simulink model "obstacle_detection"  (R2022b)
settings: Solver=VariableStepAuto  StartTime=0.0  StopTime=10.0  RelTol=1e-3
values from neighbouring files (symbols this model uses):
  m = 12    [mpc.m]    (also in mpc_soln.m; qp_soln.m)
  N = 50    [mpc.m]    (also in mpc_caller.m = 20; qp_caller.m = params.N)
  X = [p; reshape(R, [9 1]); v; R'*w]    [mpc_caller.m]    (also in qp_caller.m)
undefined symbols (not defined in the file or in its folder): Y, Z
libraries: sm_lib x269, nesl_utility x117, simulink x2
(part 4 of 5)

== system obstacle_detection/Subsystem11 ==
  PS-Simulink Converter : nesl_utility/PS-Simulink Converter  PhysicalDomain=network_engine_domain  SubClassName=ps_output  LeftPortType=input  RightPortType=output  PseudoPeriodic=off  Frequencies=[]  VectorFormat=inherit  Unit=inherit  AffineConversion=off
  PS-Simulink Converter1 : nesl_utility/PS-Simulink Converter  PhysicalDomain=network_engine_domain  SubClassName=ps_output  LeftPortType=input  RightPortType=output  PseudoPeriodic=off  Frequencies=[]  VectorFormat=inherit  Unit=inherit  AffineConversion=off
  PS-Simulink Converter2 : nesl_utility/PS-Simulink Converter  PhysicalDomain=network_engine_domain  SubClassName=ps_output  LeftPortType=input  RightPortType=output  PseudoPeriodic=off  Frequencies=[]  VectorFormat=inherit  Unit=inherit  AffineConversion=off
  1 : PMIOPort  Side=Left
  2 : PMIOPort  Port=2  Side=Left
  3 : PMIOPort  Port=3  Side=Left
  q : Outport
  w : Outport  Port=2
  t : Outport  Port=3
  wires:
  PS-Simulink Converter2/1 -> t/1
  PS-Simulink Converter1/1 -> w/1
  PS-Simulink Converter/1 -> q/1
  connections:
  3/RConn1 -- PS-Simulink Converter2/LConn1
  2/RConn1 -- PS-Simulink Converter1/LConn1
  1/RConn1 -- PS-Simulink Converter/LConn1

== system obstacle_detection/Subsystem12 ==
  PS-Simulink Converter : nesl_utility/PS-Simulink Converter  PhysicalDomain=network_engine_domain  SubClassName=ps_output  LeftPortType=input  RightPortType=output  PseudoPeriodic=off  Frequencies=[]  VectorFormat=inherit  Unit=inherit  AffineConversion=off
  PS-Simulink Converter1 : nesl_utility/PS-Simulink Converter  PhysicalDomain=network_engine_domain  SubClassName=ps_output  LeftPortType=input  RightPortType=output  PseudoPeriodic=off  Frequencies=[]  VectorFormat=inherit  Unit=inherit  AffineConversion=off
  PS-Simulink Converter2 : nesl_utility/PS-Simulink Converter  PhysicalDomain=network_engine_domain  SubClassName=ps_output  LeftPortType=input  RightPortType=output  PseudoPeriodic=off  Frequencies=[]  VectorFormat=inherit  Unit=inherit  AffineConversion=off
  1 : PMIOPort  Side=Left
  2 : PMIOPort  Port=2  Side=Left
  3 : PMIOPort  Port=3  Side=Left
  q : Outport
  w : Outport  Port=2
  t : Outport  Port=3
  wires:
  PS-Simulink Converter2/1 -> t/1
  PS-Simulink Converter1/1 -> w/1
  PS-Simulink Converter/1 -> q/1
  connections:
  3/RConn1 -- PS-Simulink Converter2/LConn1
  2/RConn1 -- PS-Simulink Converter1/LConn1
  1/RConn1 -- PS-Simulink Converter/LConn1

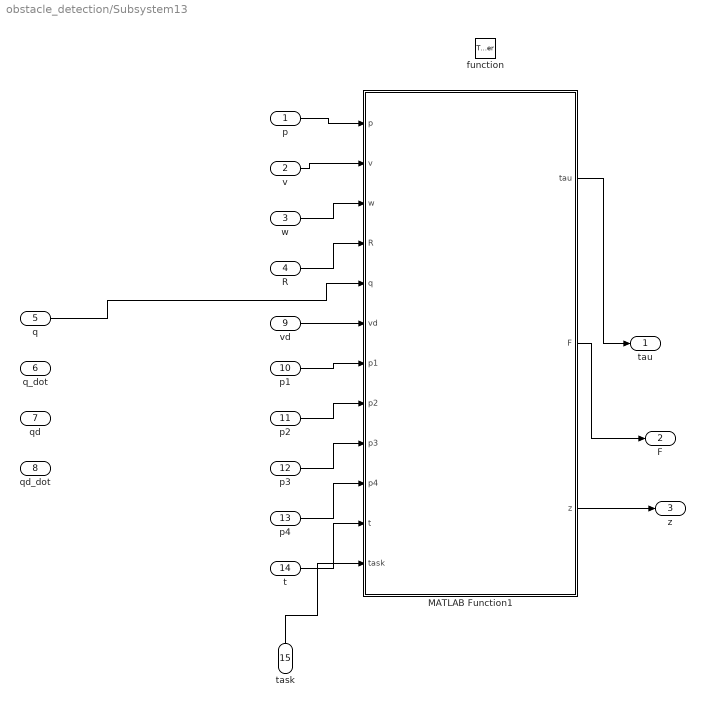
== system obstacle_detection/Subsystem13 ==
  p : Inport
  v : Inport  Port=2
  w : Inport  Port=3
  R : Inport  Port=4
  q : Inport  Port=5
  q_dot : Inport  Port=6
  qd : Inport  Port=7
  qd_dot : Inport  Port=8
  vd : Inport  Port=9
  p1 : Inport  Port=10
  p2 : Inport  Port=11
  p3 : Inport  Port=12
  p4 : Inport  Port=13
  t : Inport  Port=14
  task : Inport  Port=15
  function : TriggerPort  TriggerType=function-call  VariantControl=Variant
  MATLAB Function1 : MATLAB Function  TreatAsAtomicUnit=on
  tau : Outport
  F : Outport  Port=2
  z : Outport  Port=3
  wires:
  p/1 -> MATLAB Function1/1(p)
  v/1 -> MATLAB Function1/2(v)
  w/1 -> MATLAB Function1/3(w)
  R/1 -> MATLAB Function1/4(R)
  q/1 -> MATLAB Function1/5(q)
  p1/1 -> MATLAB Function1/7(p1)
  p2/1 -> MATLAB Function1/8(p2)
  p4/1 -> MATLAB Function1/10(p4)
  p3/1 -> MATLAB Function1/9(p3)
  t/1 -> MATLAB Function1/11(t)
  MATLAB Function1/1(tau) -> tau/1
  MATLAB Function1/2(F) -> F/1
  task/1 -> MATLAB Function1/12(task)
  vd/1 -> MATLAB Function1/6(vd)
  MATLAB Function1/3(z) -> z/1

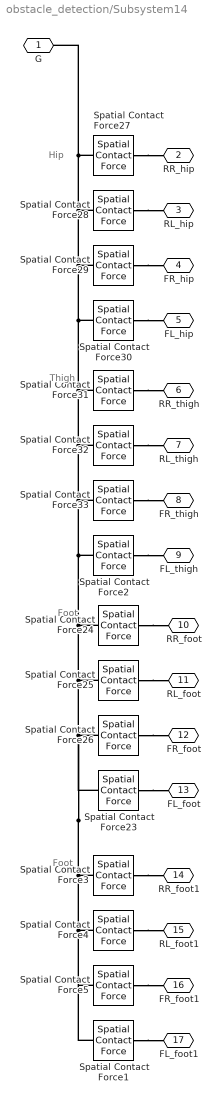
== system obstacle_detection/Subsystem14 ==
  note: Hip
  note: Foot
  note: Thigh
  note: Foot
  Spatial Contact Force{1..5,23..33} (16 alike) : sm_lib/Forces and Torques/Spatial Contact Force  SenseContactBaseRotation=off  SenseContactBaseTranslation=off  CoefficientOfDynamicFriction=1  CoefficientOfStaticFriction=1  NormalDamping=1e3  NormalDampingUnits=N/(m/s)  SenseContactSignal=off  NormalStiffness=1e6  NormalStiffnessUnits=N/m  FrictionalCriticalVelocity=1e-3  FrictionalCriticalVelocityUnits=m/s  ZeroCrossDetectContactStartAndEnd=off  SenseContactFollowerRotation=off  SenseContactFollowerTranslation=off  FrictionType=SmoothStickSlip  SenseFrictionalForceMagnitude=off  SenseNormalForceMagnitude=off  NormalForceType=SmoothSpringDamper  SenseNormalVelocity=off  SenseSeparationDistance=off  SenseTangentialVelocity=off  NormalTransitionRegionWidth=1e-4  NormalTransitionRegionWidthUnits=m
  G : PMIOPort  Side=Left
  RR_hip : PMIOPort  Port=2  Side=Right
  RL_hip : PMIOPort  Port=3  Side=Right
  FR_hip : PMIOPort  Port=4  Side=Right
  FL_hip : PMIOPort  Port=5  Side=Right
  RR_thigh : PMIOPort  Port=6  Side=Right
  RL_thigh : PMIOPort  Port=7  Side=Right
  FR_thigh : PMIOPort  Port=8  Side=Right
  FL_thigh : PMIOPort  Port=9  Side=Right
  RR_foot : PMIOPort  Port=10  Side=Right
  RL_foot : PMIOPort  Port=11  Side=Right
  FR_foot : PMIOPort  Port=12  Side=Right
  FL_foot : PMIOPort  Port=13  Side=Right
  RR_foot1 : PMIOPort  Port=14  Side=Right
  RL_foot1 : PMIOPort  Port=15  Side=Right
  FR_foot1 : PMIOPort  Port=16  Side=Right
  FL_foot1 : PMIOPort  Port=17  Side=Right
  connections:
  Spatial Contact Force29/RConn1 -- FR_hip/RConn1
  Spatial Contact Force23/RConn1 -- FL_foot/RConn1
  Spatial Contact Force24/RConn1 -- RR_foot/RConn1
  Spatial Contact Force32/RConn1 -- RL_thigh/RConn1
  Spatial Contact Force33/RConn1 -- FR_thigh/RConn1
  Spatial Contact Force30/RConn1 -- FL_hip/RConn1
  Spatial Contact Force25/RConn1 -- RL_foot/RConn1
  Spatial Contact Force2/RConn1 -- FL_thigh/RConn1
  Spatial Contact Force27/RConn1 -- RR_hip/RConn1
  Spatial Contact Force28/RConn1 -- RL_hip/RConn1
  Spatial Contact Force26/RConn1 -- FR_foot/RConn1
  Spatial Contact Force31/RConn1 -- RR_thigh/RConn1
  Spatial Contact Force25/LConn1 -- Spatial Contact Force23/LConn1 -- Spatial Contact Force3/LConn1 -- Spatial Contact Force4/LConn1 -- Spatial Contact Force1/LConn1 -- Spatial Contact Force5/LConn1 -- Spatial Contact Force26/LConn1 -- Spatial Contact Force24/LConn1 -- Spatial Contact Force2/LConn1 -- Spatial Contact Force33/LConn1 -- Spatial Contact Force32/LConn1 -- Spatial Contact Force31/LConn1 -- Spatial Contact Force30/LConn1 -- Spatial Contact Force29/LConn1 -- Spatial Contact Force28/LConn1 -- Spatial Contact Force27/LConn1 -- G/RConn1
  Spatial Contact Force3/RConn1 -- RR_foot1/RConn1
  Spatial Contact Force1/RConn1 -- FL_foot1/RConn1
  Spatial Contact Force4/RConn1 -- RL_foot1/RConn1
  Spatial Contact Force5/RConn1 -- FR_foot1/RConn1

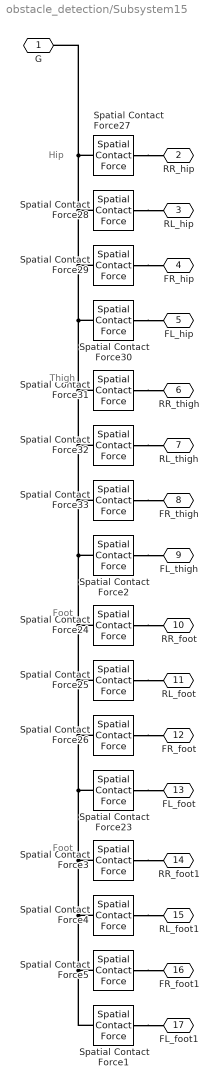
== system obstacle_detection/Subsystem15 ==
  note: Hip
  note: Foot
  note: Thigh
  note: Foot
  Spatial Contact Force{1..5,23..33} (16 alike) : sm_lib/Forces and Torques/Spatial Contact Force  SenseContactBaseRotation=off  SenseContactBaseTranslation=off  CoefficientOfDynamicFriction=1  CoefficientOfStaticFriction=1  NormalDamping=1e3  NormalDampingUnits=N/(m/s)  SenseContactSignal=off  NormalStiffness=1e6  NormalStiffnessUnits=N/m  FrictionalCriticalVelocity=1e-3  FrictionalCriticalVelocityUnits=m/s  ZeroCrossDetectContactStartAndEnd=off  SenseContactFollowerRotation=off  SenseContactFollowerTranslation=off  FrictionType=SmoothStickSlip  SenseFrictionalForceMagnitude=off  SenseNormalForceMagnitude=off  NormalForceType=SmoothSpringDamper  SenseNormalVelocity=off  SenseSeparationDistance=off  SenseTangentialVelocity=off  NormalTransitionRegionWidth=1e-4  NormalTransitionRegionWidthUnits=m
  G : PMIOPort  Side=Left
  RR_hip : PMIOPort  Port=2  Side=Right
  RL_hip : PMIOPort  Port=3  Side=Right
  FR_hip : PMIOPort  Port=4  Side=Right
  FL_hip : PMIOPort  Port=5  Side=Right
  RR_thigh : PMIOPort  Port=6  Side=Right
  RL_thigh : PMIOPort  Port=7  Side=Right
  FR_thigh : PMIOPort  Port=8  Side=Right
  FL_thigh : PMIOPort  Port=9  Side=Right
  RR_foot : PMIOPort  Port=10  Side=Right
  RL_foot : PMIOPort  Port=11  Side=Right
  FR_foot : PMIOPort  Port=12  Side=Right
  FL_foot : PMIOPort  Port=13  Side=Right
  RR_foot1 : PMIOPort  Port=14  Side=Right
  RL_foot1 : PMIOPort  Port=15  Side=Right
  FR_foot1 : PMIOPort  Port=16  Side=Right
  FL_foot1 : PMIOPort  Port=17  Side=Right
  connections:
  Spatial Contact Force29/RConn1 -- FR_hip/RConn1
  Spatial Contact Force5/LConn1 -- Spatial Contact Force1/LConn1 -- Spatial Contact Force4/LConn1 -- Spatial Contact Force26/LConn1 -- Spatial Contact Force25/LConn1 -- Spatial Contact Force24/LConn1 -- Spatial Contact Force2/LConn1 -- Spatial Contact Force33/LConn1 -- Spatial Contact Force27/LConn1 -- G/RConn1 -- Spatial Contact Force28/LConn1 -- Spatial Contact Force29/LConn1 -- Spatial Contact Force30/LConn1 -- Spatial Contact Force31/LConn1 -- Spatial Contact Force32/LConn1 -- Spatial Contact Force23/LConn1 -- Spatial Contact Force3/LConn1
  Spatial Contact Force23/RConn1 -- FL_foot/RConn1
  Spatial Contact Force24/RConn1 -- RR_foot/RConn1
  Spatial Contact Force32/RConn1 -- RL_thigh/RConn1
  Spatial Contact Force33/RConn1 -- FR_thigh/RConn1
  Spatial Contact Force30/RConn1 -- FL_hip/RConn1
  Spatial Contact Force25/RConn1 -- RL_foot/RConn1
  Spatial Contact Force2/RConn1 -- FL_thigh/RConn1
  Spatial Contact Force27/RConn1 -- RR_hip/RConn1
  Spatial Contact Force28/RConn1 -- RL_hip/RConn1
  Spatial Contact Force26/RConn1 -- FR_foot/RConn1
  Spatial Contact Force31/RConn1 -- RR_thigh/RConn1
  Spatial Contact Force1/RConn1 -- FL_foot1/RConn1
  Spatial Contact Force4/RConn1 -- RL_foot1/RConn1
  Spatial Contact Force3/RConn1 -- RR_foot1/RConn1
  Spatial Contact Force5/RConn1 -- FR_foot1/RConn1

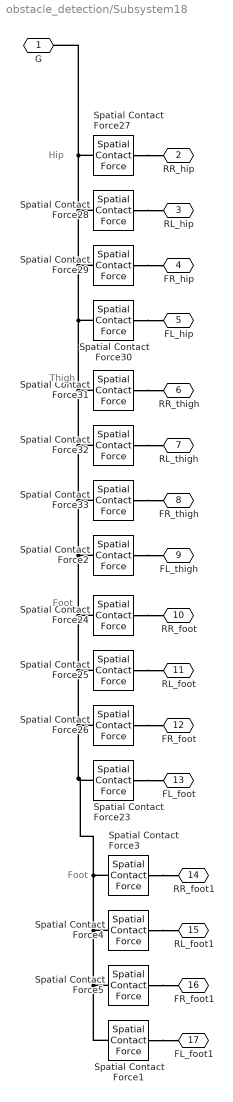
== system obstacle_detection/Subsystem18 ==
  note: Thigh
  note: Foot
  note: Hip
  note: Foot
  Spatial Contact Force{1..5,23..33} (16 alike) : sm_lib/Forces and Torques/Spatial Contact Force  SenseContactBaseRotation=off  SenseContactBaseTranslation=off  CoefficientOfDynamicFriction=1  CoefficientOfStaticFriction=1  NormalDamping=1e3  NormalDampingUnits=N/(m/s)  SenseContactSignal=off  NormalStiffness=1e6  NormalStiffnessUnits=N/m  FrictionalCriticalVelocity=1e-3  FrictionalCriticalVelocityUnits=m/s  ZeroCrossDetectContactStartAndEnd=off  SenseContactFollowerRotation=off  SenseContactFollowerTranslation=off  FrictionType=SmoothStickSlip  SenseFrictionalForceMagnitude=off  SenseNormalForceMagnitude=off  NormalForceType=SmoothSpringDamper  SenseNormalVelocity=off  SenseSeparationDistance=off  SenseTangentialVelocity=off  NormalTransitionRegionWidth=1e-4  NormalTransitionRegionWidthUnits=m
  G : PMIOPort  Side=Left
  RR_hip : PMIOPort  Port=2  Side=Right
  RL_hip : PMIOPort  Port=3  Side=Right
  FR_hip : PMIOPort  Port=4  Side=Right
  FL_hip : PMIOPort  Port=5  Side=Right
  RR_thigh : PMIOPort  Port=6  Side=Right
  RL_thigh : PMIOPort  Port=7  Side=Right
  FR_thigh : PMIOPort  Port=8  Side=Right
  FL_thigh : PMIOPort  Port=9  Side=Right
  RR_foot : PMIOPort  Port=10  Side=Right
  RL_foot : PMIOPort  Port=11  Side=Right
  FR_foot : PMIOPort  Port=12  Side=Right
  FL_foot : PMIOPort  Port=13  Side=Right
  RR_foot1 : PMIOPort  Port=14  Side=Right
  RL_foot1 : PMIOPort  Port=15  Side=Right
  FR_foot1 : PMIOPort  Port=16  Side=Right
  FL_foot1 : PMIOPort  Port=17  Side=Right
  connections:
  Spatial Contact Force31/RConn1 -- RR_thigh/RConn1
  Spatial Contact Force26/RConn1 -- FR_foot/RConn1
  Spatial Contact Force28/RConn1 -- RL_hip/RConn1
  Spatial Contact Force27/RConn1 -- RR_hip/RConn1
  Spatial Contact Force2/RConn1 -- FL_thigh/RConn1
  Spatial Contact Force25/RConn1 -- RL_foot/RConn1
  Spatial Contact Force30/RConn1 -- FL_hip/RConn1
  Spatial Contact Force33/RConn1 -- FR_thigh/RConn1
  Spatial Contact Force32/RConn1 -- RL_thigh/RConn1
  Spatial Contact Force24/RConn1 -- RR_foot/RConn1
  Spatial Contact Force23/RConn1 -- FL_foot/RConn1
  Spatial Contact Force29/RConn1 -- FR_hip/RConn1
  Spatial Contact Force3/LConn1 -- Spatial Contact Force26/LConn1 -- Spatial Contact Force25/LConn1 -- Spatial Contact Force33/LConn1 -- Spatial Contact Force32/LConn1 -- G/RConn1 -- Spatial Contact Force27/LConn1 -- Spatial Contact Force28/LConn1 -- Spatial Contact Force29/LConn1 -- Spatial Contact Force30/LConn1 -- Spatial Contact Force31/LConn1 -- Spatial Contact Force2/LConn1 -- Spatial Contact Force24/LConn1 -- Spatial Contact Force23/LConn1 -- Spatial Contact Force4/LConn1 -- Spatial Contact Force1/LConn1 -- Spatial Contact Force5/LConn1
  Spatial Contact Force4/RConn1 -- RL_foot1/RConn1
  Spatial Contact Force1/RConn1 -- FL_foot1/RConn1
  Spatial Contact Force3/RConn1 -- RR_foot1/RConn1
  Spatial Contact Force5/RConn1 -- FR_foot1/RConn1

== system obstacle_detection/Subsystem2 ==
  PS-Simulink Converter : nesl_utility/PS-Simulink Converter  PhysicalDomain=network_engine_domain  SubClassName=ps_output  LeftPortType=input  RightPortType=output  PseudoPeriodic=off  Frequencies=[]  VectorFormat=inherit  Unit=inherit  AffineConversion=off
  PS-Simulink Converter1 : nesl_utility/PS-Simulink Converter  PhysicalDomain=network_engine_domain  SubClassName=ps_output  LeftPortType=input  RightPortType=output  PseudoPeriodic=off  Frequencies=[]  VectorFormat=inherit  Unit=inherit  AffineConversion=off
  PS-Simulink Converter2 : nesl_utility/PS-Simulink Converter  PhysicalDomain=network_engine_domain  SubClassName=ps_output  LeftPortType=input  RightPortType=output  PseudoPeriodic=off  Frequencies=[]  VectorFormat=inherit  Unit=inherit  AffineConversion=off
  1 : PMIOPort  Side=Left
  2 : PMIOPort  Port=2  Side=Left
  3 : PMIOPort  Port=3  Side=Left
  q : Outport
  w : Outport  Port=2
  t : Outport  Port=3
  wires:
  PS-Simulink Converter2/1 -> t/1
  PS-Simulink Converter1/1 -> w/1
  PS-Simulink Converter/1 -> q/1
  connections:
  3/RConn1 -- PS-Simulink Converter2/LConn1
  2/RConn1 -- PS-Simulink Converter1/LConn1
  1/RConn1 -- PS-Simulink Converter/LConn1

== system obstacle_detection/Subsystem3 ==
  PS-Simulink Converter : nesl_utility/PS-Simulink Converter  PhysicalDomain=network_engine_domain  SubClassName=ps_output  LeftPortType=input  RightPortType=output  PseudoPeriodic=off  Frequencies=[]  VectorFormat=inherit  Unit=inherit  AffineConversion=off
  PS-Simulink Converter1 : nesl_utility/PS-Simulink Converter  PhysicalDomain=network_engine_domain  SubClassName=ps_output  LeftPortType=input  RightPortType=output  PseudoPeriodic=off  Frequencies=[]  VectorFormat=inherit  Unit=inherit  AffineConversion=off
  PS-Simulink Converter2 : nesl_utility/PS-Simulink Converter  PhysicalDomain=network_engine_domain  SubClassName=ps_output  LeftPortType=input  RightPortType=output  PseudoPeriodic=off  Frequencies=[]  VectorFormat=inherit  Unit=inherit  AffineConversion=off
  1 : PMIOPort  Side=Left
  2 : PMIOPort  Port=2  Side=Left
  3 : PMIOPort  Port=3  Side=Left
  q : Outport
  w : Outport  Port=2
  t : Outport  Port=3
  wires:
  PS-Simulink Converter2/1 -> t/1
  PS-Simulink Converter1/1 -> w/1
  PS-Simulink Converter/1 -> q/1
  connections:
  3/RConn1 -- PS-Simulink Converter2/LConn1
  2/RConn1 -- PS-Simulink Converter1/LConn1
  1/RConn1 -- PS-Simulink Converter/LConn1

== system obstacle_detection/Subsystem4 ==
  PS-Simulink Converter : nesl_utility/PS-Simulink Converter  PhysicalDomain=network_engine_domain  SubClassName=ps_output  LeftPortType=input  RightPortType=output  PseudoPeriodic=off  Frequencies=[]  VectorFormat=inherit  Unit=inherit  AffineConversion=off
  PS-Simulink Converter1 : nesl_utility/PS-Simulink Converter  PhysicalDomain=network_engine_domain  SubClassName=ps_output  LeftPortType=input  RightPortType=output  PseudoPeriodic=off  Frequencies=[]  VectorFormat=inherit  Unit=inherit  AffineConversion=off
  PS-Simulink Converter2 : nesl_utility/PS-Simulink Converter  PhysicalDomain=network_engine_domain  SubClassName=ps_output  LeftPortType=input  RightPortType=output  PseudoPeriodic=off  Frequencies=[]  VectorFormat=inherit  Unit=inherit  AffineConversion=off
  1 : PMIOPort  Side=Left
  2 : PMIOPort  Port=2  Side=Left
  3 : PMIOPort  Port=3  Side=Left
  q : Outport
  w : Outport  Port=2
  t : Outport  Port=3
  wires:
  PS-Simulink Converter/1 -> q/1
  PS-Simulink Converter1/1 -> w/1
  PS-Simulink Converter2/1 -> t/1
  connections:
  1/RConn1 -- PS-Simulink Converter/LConn1
  2/RConn1 -- PS-Simulink Converter1/LConn1
  3/RConn1 -- PS-Simulink Converter2/LConn1

== system obstacle_detection/Subsystem5 ==
  PS-Simulink Converter : nesl_utility/PS-Simulink Converter  PhysicalDomain=network_engine_domain  SubClassName=ps_output  LeftPortType=input  RightPortType=output  PseudoPeriodic=off  Frequencies=[]  VectorFormat=inherit  Unit=inherit  AffineConversion=off
  PS-Simulink Converter1 : nesl_utility/PS-Simulink Converter  PhysicalDomain=network_engine_domain  SubClassName=ps_output  LeftPortType=input  RightPortType=output  PseudoPeriodic=off  Frequencies=[]  VectorFormat=inherit  Unit=inherit  AffineConversion=off
  PS-Simulink Converter2 : nesl_utility/PS-Simulink Converter  PhysicalDomain=network_engine_domain  SubClassName=ps_output  LeftPortType=input  RightPortType=output  PseudoPeriodic=off  Frequencies=[]  VectorFormat=inherit  Unit=inherit  AffineConversion=off
  1 : PMIOPort  Side=Left
  2 : PMIOPort  Port=2  Side=Left
  3 : PMIOPort  Port=3  Side=Left
  q : Outport
  w : Outport  Port=2
  t : Outport  Port=3
  wires:
  PS-Simulink Converter/1 -> q/1
  PS-Simulink Converter1/1 -> w/1
  PS-Simulink Converter2/1 -> t/1
  connections:
  1/RConn1 -- PS-Simulink Converter/LConn1
  2/RConn1 -- PS-Simulink Converter1/LConn1
  3/RConn1 -- PS-Simulink Converter2/LConn1

== system obstacle_detection/Subsystem6 ==
  PS-Simulink Converter : nesl_utility/PS-Simulink Converter  PhysicalDomain=network_engine_domain  SubClassName=ps_output  LeftPortType=input  RightPortType=output  PseudoPeriodic=off  Frequencies=[]  VectorFormat=inherit  Unit=inherit  AffineConversion=off
  PS-Simulink Converter1 : nesl_utility/PS-Simulink Converter  PhysicalDomain=network_engine_domain  SubClassName=ps_output  LeftPortType=input  RightPortType=output  PseudoPeriodic=off  Frequencies=[]  VectorFormat=inherit  Unit=inherit  AffineConversion=off
  PS-Simulink Converter2 : nesl_utility/PS-Simulink Converter  PhysicalDomain=network_engine_domain  SubClassName=ps_output  LeftPortType=input  RightPortType=output  PseudoPeriodic=off  Frequencies=[]  VectorFormat=inherit  Unit=inherit  AffineConversion=off
  1 : PMIOPort  Side=Left
  2 : PMIOPort  Port=2  Side=Left
  3 : PMIOPort  Port=3  Side=Left
  q : Outport
  w : Outport  Port=2
  t : Outport  Port=3
  wires:
  PS-Simulink Converter/1 -> q/1
  PS-Simulink Converter1/1 -> w/1
  PS-Simulink Converter2/1 -> t/1
  connections:
  1/RConn1 -- PS-Simulink Converter/LConn1
  2/RConn1 -- PS-Simulink Converter1/LConn1
  3/RConn1 -- PS-Simulink Converter2/LConn1

== system obstacle_detection/Subsystem7 ==
  PS-Simulink Converter : nesl_utility/PS-Simulink Converter  PhysicalDomain=network_engine_domain  SubClassName=ps_output  LeftPortType=input  RightPortType=output  PseudoPeriodic=off  Frequencies=[]  VectorFormat=inherit  Unit=inherit  AffineConversion=off
  PS-Simulink Converter1 : nesl_utility/PS-Simulink Converter  PhysicalDomain=network_engine_domain  SubClassName=ps_output  LeftPortType=input  RightPortType=output  PseudoPeriodic=off  Frequencies=[]  VectorFormat=inherit  Unit=inherit  AffineConversion=off
  PS-Simulink Converter2 : nesl_utility/PS-Simulink Converter  PhysicalDomain=network_engine_domain  SubClassName=ps_output  LeftPortType=input  RightPortType=output  PseudoPeriodic=off  Frequencies=[]  VectorFormat=inherit  Unit=inherit  AffineConversion=off
  1 : PMIOPort  Side=Left
  2 : PMIOPort  Port=2  Side=Left
  3 : PMIOPort  Port=3  Side=Left
  q : Outport
  w : Outport  Port=2
  t : Outport  Port=3
  wires:
  PS-Simulink Converter2/1 -> t/1
  PS-Simulink Converter1/1 -> w/1
  PS-Simulink Converter/1 -> q/1
  connections:
  3/RConn1 -- PS-Simulink Converter2/LConn1
  2/RConn1 -- PS-Simulink Converter1/LConn1
  1/RConn1 -- PS-Simulink Converter/LConn1

== system obstacle_detection/Subsystem8 ==
  PS-Simulink Converter : nesl_utility/PS-Simulink Converter  PhysicalDomain=network_engine_domain  SubClassName=ps_output  LeftPortType=input  RightPortType=output  PseudoPeriodic=off  Frequencies=[]  VectorFormat=inherit  Unit=inherit  AffineConversion=off
  PS-Simulink Converter1 : nesl_utility/PS-Simulink Converter  PhysicalDomain=network_engine_domain  SubClassName=ps_output  LeftPortType=input  RightPortType=output  PseudoPeriodic=off  Frequencies=[]  VectorFormat=inherit  Unit=inherit  AffineConversion=off
  PS-Simulink Converter2 : nesl_utility/PS-Simulink Converter  PhysicalDomain=network_engine_domain  SubClassName=ps_output  LeftPortType=input  RightPortType=output  PseudoPeriodic=off  Frequencies=[]  VectorFormat=inherit  Unit=inherit  AffineConversion=off
  1 : PMIOPort  Side=Left
  2 : PMIOPort  Port=2  Side=Left
  3 : PMIOPort  Port=3  Side=Left
  q : Outport
  w : Outport  Port=2
  t : Outport  Port=3
  wires:
  PS-Simulink Converter2/1 -> t/1
  PS-Simulink Converter1/1 -> w/1
  PS-Simulink Converter/1 -> q/1
  connections:
  3/RConn1 -- PS-Simulink Converter2/LConn1
  2/RConn1 -- PS-Simulink Converter1/LConn1
  1/RConn1 -- PS-Simulink Converter/LConn1

== system obstacle_detection/Subsystem9 ==
  PS-Simulink Converter : nesl_utility/PS-Simulink Converter  PhysicalDomain=network_engine_domain  SubClassName=ps_output  LeftPortType=input  RightPortType=output  PseudoPeriodic=off  Frequencies=[]  VectorFormat=inherit  Unit=inherit  AffineConversion=off
  PS-Simulink Converter1 : nesl_utility/PS-Simulink Converter  PhysicalDomain=network_engine_domain  SubClassName=ps_output  LeftPortType=input  RightPortType=output  PseudoPeriodic=off  Frequencies=[]  VectorFormat=inherit  Unit=inherit  AffineConversion=off
  PS-Simulink Converter2 : nesl_utility/PS-Simulink Converter  PhysicalDomain=network_engine_domain  SubClassName=ps_output  LeftPortType=input  RightPortType=output  PseudoPeriodic=off  Frequencies=[]  VectorFormat=inherit  Unit=inherit  AffineConversion=off
  1 : PMIOPort  Side=Left
  2 : PMIOPort  Port=2  Side=Left
  3 : PMIOPort  Port=3  Side=Left
  q : Outport
  w : Outport  Port=2
  t : Outport  Port=3
  wires:
  PS-Simulink Converter2/1 -> t/1
  PS-Simulink Converter1/1 -> w/1
  PS-Simulink Converter/1 -> q/1
  connections:
  3/RConn1 -- PS-Simulink Converter2/LConn1
  2/RConn1 -- PS-Simulink Converter1/LConn1
  1/RConn1 -- PS-Simulink Converter/LConn1

== system obstacle_detection/base ==
  ReferenceFrame : sm_lib/Frames and Transforms/Reference Frame
  Visual : sm_lib/Body Elements/Brick Solid  GraphicAmbientColor=[0.15 0.15 0.15 1.0]  BasedOnType=Density  BrickDimensions=[0.001, 0.001, 0.001]  BrickDimensionUnits=m  CenterOfMass=[0, 0, 0]  CenterOfMassUnits=m  GraphicDiffuseColor=[0.5, 0.5, 0.5]  Density=1000  DensityUnits=kg/m^3  DoExposeReferenceFrame=on  GraphicEmissiveColor=[0.0 0.0 0.0 1.0]  ExportEntireGeometry=off  SerializedFrames=<Frames/>  MarkerShape=Sphere  MarkerSize=10  GraphicType=FromGeometry  InertiaType=Custom  Mass=0  MassUnits=kg  MomentsOfInertia=[0, 0, 0]  MomentsOfInertiaUnits=kg*m^2  GraphicOpacity=1  ProductsOfInertia=[0, 0, 0]  ProductsOfInertiaUnits=kg*m^2  GraphicShininess=75  GraphicSpecularColor=[0.5 0.5 0.5 1.0]  GraphicVisPropType=SimpleVisualProperties
  VisualOriginTransform : sm_lib/Frames and Transforms/Rigid Transform  TranslationMethod=Cartesian  TranslationStandardOffset=0  TranslationLengthUnit=m  TranslationStandardAxis=+Z  TranslationCartesianOffset=[0, 0, 0]  TranslationROffset=0  TranslationROffsetUnits=m  TranslationZOffset=0  TranslationZOffsetUnits=m  TranslationThetaOffset=0  TranslationThetaOffsetUnits=deg  RotationMethod=RotationSequence  RotationAngleUnits=deg  RotationStandardAxis=+Z  RotationAngle=0.0  RotationArbitraryAxis=[0 0 1]  FollAlignAxisA=+X  BaseAlignAxisA=+Y  FollAlignAxisB=+Y  BaseAlignAxisB=+Z  RotationSequenceAxes=BaseAxes  RotationSequence=XYZ  RotationSequenceAngles=[0, 0, 0]  RotationSequenceAnglesUnits=rad  RotationMatrix=[1 0 0; 0 1 0; 0 0 1]  Quaternion=[1 0 0 0]
  floating_base_OriginTransform : sm_lib/Frames and Transforms/Rigid Transform  TranslationMethod=Cartesian  TranslationStandardOffset=0  TranslationLengthUnit=m  TranslationStandardAxis=+Z  TranslationCartesianOffset=[0, 0, 0]  TranslationROffset=0  TranslationROffsetUnits=m  TranslationZOffset=0  TranslationZOffsetUnits=m  TranslationThetaOffset=0  TranslationThetaOffsetUnits=deg  RotationMethod=RotationSequence  RotationAngleUnits=deg  RotationStandardAxis=+Z  RotationAngle=0.0  RotationArbitraryAxis=[0 0 1]  FollAlignAxisA=+X  BaseAlignAxisA=+Y  FollAlignAxisB=+Y  BaseAlignAxisB=+Z  RotationSequenceAxes=BaseAxes  RotationSequence=XYZ  RotationSequenceAngles=[0, 0, 0]  RotationSequenceAnglesUnits=rad  RotationMatrix=[1 0 0; 0 1 0; 0 0 1]  Quaternion=[1 0 0 0]
  F : PMIOPort  Side=Left
  F1 : PMIOPort  Port=2  Side=Right
  connections:
  VisualOriginTransform/LConn1 -- ReferenceFrame/RConn1 -- F/RConn1 -- floating_base_OriginTransform/LConn1
  Visual/RConn1 -- VisualOriginTransform/RConn1
  floating_base_OriginTransform/RConn1 -- F1/RConn1

== system obstacle_detection/imu_link ==
  Inertia : sm_lib/Body Elements/Inertia  InertiaType=Custom  Mass=0.001  MassUnits=kg  CenterOfMass=[0, 0, 0]  CenterOfMassUnits=m  MomentsOfInertia=[0.0001, 0.0001, 0.0001]  MomentsOfInertiaUnits=kg*m^2  ProductsOfInertia=[0, 0, 0]  ProductsOfInertiaUnits=kg*m^2  GraphicType=None  MarkerShape=Inertia  MarkerSize=20  GraphicVisPropType=SimpleVisualProperties  GraphicDiffuseColor=[0.5 0.5 0.5]  GraphicSpecularColor=[0.5 0.5 0.5 1.0]  GraphicAmbientColor=[0.15 0.15 0.15 1.0]  GraphicEmissiveColor=[0.0 0.0 0.0 1.0]  GraphicShininess=75  GraphicOpacity=1.0
  InertiaOriginTransform : sm_lib/Frames and Transforms/Rigid Transform  TranslationMethod=Cartesian  TranslationStandardOffset=0  TranslationLengthUnit=m  TranslationStandardAxis=+Z  TranslationCartesianOffset=[0, 0, 0]  TranslationROffset=0  TranslationROffsetUnits=m  TranslationZOffset=0  TranslationZOffsetUnits=m  TranslationThetaOffset=0  TranslationThetaOffsetUnits=deg  RotationMethod=RotationSequence  RotationAngleUnits=deg  RotationStandardAxis=+Z  RotationAngle=0.0  RotationArbitraryAxis=[0 0 1]  FollAlignAxisA=+X  BaseAlignAxisA=+Y  FollAlignAxisB=+Y  BaseAlignAxisB=+Z  RotationSequenceAxes=BaseAxes  RotationSequence=XYZ  RotationSequenceAngles=[0, 0, 0]  RotationSequenceAnglesUnits=rad  RotationMatrix=[1 0 0; 0 1 0; 0 0 1]  Quaternion=[1 0 0 0]
  ReferenceFrame : sm_lib/Frames and Transforms/Reference Frame
  Visual : sm_lib/Body Elements/Brick Solid  GraphicAmbientColor=[0.15 0.15 0.15 1.0]  BasedOnType=Density  BrickDimensions=[0.001, 0.001, 0.001]  BrickDimensionUnits=m  CenterOfMass=[0, 0, 0]  CenterOfMassUnits=m  GraphicDiffuseColor=[0.8, 0, 0]  Density=1000  DensityUnits=kg/m^3  DoExposeReferenceFrame=on  GraphicEmissiveColor=[0.0 0.0 0.0 1.0]  ExportEntireGeometry=off  SerializedFrames=<Frames/>  MarkerShape=Sphere  MarkerSize=10  GraphicType=FromGeometry  InertiaType=Custom  Mass=0  MassUnits=kg  MomentsOfInertia=[0, 0, 0]  MomentsOfInertiaUnits=kg*m^2  GraphicOpacity=1  ProductsOfInertia=[0, 0, 0]  ProductsOfInertiaUnits=kg*m^2  GraphicShininess=75  GraphicSpecularColor=[0.5 0.5 0.5 1.0]  GraphicVisPropType=SimpleVisualProperties
  VisualOriginTransform : sm_lib/Frames and Transforms/Rigid Transform  TranslationMethod=Cartesian  TranslationStandardOffset=0  TranslationLengthUnit=m  TranslationStandardAxis=+Z  TranslationCartesianOffset=[0, 0, 0]  TranslationROffset=0  TranslationROffsetUnits=m  TranslationZOffset=0  TranslationZOffsetUnits=m  TranslationThetaOffset=0  TranslationThetaOffsetUnits=deg  RotationMethod=RotationSequence  RotationAngleUnits=deg  RotationStandardAxis=+Z  RotationAngle=0.0  RotationArbitraryAxis=[0 0 1]  FollAlignAxisA=+X  BaseAlignAxisA=+Y  FollAlignAxisB=+Y  BaseAlignAxisB=+Z  RotationSequenceAxes=BaseAxes  RotationSequence=XYZ  RotationSequenceAngles=[0, 0, 0]  RotationSequenceAnglesUnits=rad  RotationMatrix=[1 0 0; 0 1 0; 0 0 1]  Quaternion=[1 0 0 0]
  F : PMIOPort  Side=Left
  connections:
  Inertia/RConn1 -- InertiaOriginTransform/RConn1
  ReferenceFrame/RConn1 -- InertiaOriginTransform/LConn1 -- VisualOriginTransform/LConn1 -- F/RConn1
  Visual/RConn1 -- VisualOriginTransform/RConn1

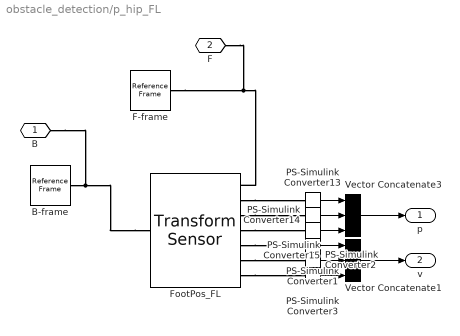
== system obstacle_detection/p_hip_FL ==
  B-frame : sm_lib/Frames and Transforms/Reference Frame
  F-frame : sm_lib/Frames and Transforms/Reference Frame
  FootPos_FL : sm_lib/Frames and Transforms/Transform Sensor  MeasurementFrame=World  SenseAngle=off  SenseAxis=off  SenseQ=off  SenseR=off  SenseRotationSequence=off  RotationSequence=XYX  SenseOmegaX=off  SenseOmegaY=off  SenseOmegaZ=off  SenseQDot=off  SenseRDot=off  SenseAlphaX=off  SenseAlphaY=off  SenseAlphaZ=off  SenseQDDot=off  SenseRDDot=off  SenseX=on  SenseY=on  SenseZ=on  SenseRad=off  SenseAzim=off  SenseDist=off  SenseInc=off  SenseXDot=on  SenseYDot=on  SenseZDot=on  SenseRadDot=off  SenseAzimDot=off  SenseDistDot=off  SenseIncDot=off  SenseXDDot=off  SenseYDDot=off  SenseZDDot=off  SenseRadDDot=off  SenseAzimDDot=off  SenseDistDDot=off  SenseIncDDot=off
  PS-Simulink Converter{1..3,13..15} (6 alike) : nesl_utility/PS-Simulink Converter  PhysicalDomain=network_engine_domain  SubClassName=ps_output  LeftPortType=input  RightPortType=output  PseudoPeriodic=off  Frequencies=[]  VectorFormat=inherit  Unit=inherit  AffineConversion=off
  Vector Concatenate1 : Concatenate  NumInputs=3
  Vector Concatenate3 : Concatenate  NumInputs=3
  B : PMIOPort  Side=Left
  F : PMIOPort  Port=2  Side=Left
  p : Outport
  v : Outport  Port=2
  wires:
  PS-Simulink Converter13/1 -> Vector Concatenate3/1
  PS-Simulink Converter15/1 -> Vector Concatenate3/3
  PS-Simulink Converter14/1 -> Vector Concatenate3/2
  Vector Concatenate3/1 -> p/1
  PS-Simulink Converter2/1 -> Vector Concatenate1/2
  PS-Simulink Converter3/1 -> Vector Concatenate1/3
  PS-Simulink Converter1/1 -> Vector Concatenate1/1
  Vector Concatenate1/1 -> v/1
  connections:
  FootPos_FL/LConn1 -- B-frame/RConn1 -- B/RConn1
  FootPos_FL/RConn1 -- F-frame/RConn1 -- F/RConn1
  FootPos_FL/RConn4 -- PS-Simulink Converter15/LConn1
  FootPos_FL/RConn2 -- PS-Simulink Converter13/LConn1
  FootPos_FL/RConn3 -- PS-Simulink Converter14/LConn1
  FootPos_FL/RConn6 -- PS-Simulink Converter2/LConn1
  FootPos_FL/RConn5 -- PS-Simulink Converter1/LConn1
  FootPos_FL/RConn7 -- PS-Simulink Converter3/LConn1

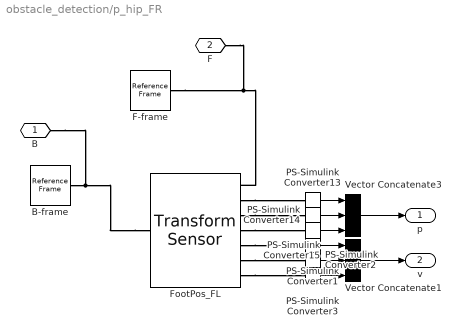
== system obstacle_detection/p_hip_FR ==
  B-frame : sm_lib/Frames and Transforms/Reference Frame
  F-frame : sm_lib/Frames and Transforms/Reference Frame
  FootPos_FL : sm_lib/Frames and Transforms/Transform Sensor  MeasurementFrame=World  SenseAngle=off  SenseAxis=off  SenseQ=off  SenseR=off  SenseRotationSequence=off  RotationSequence=XYX  SenseOmegaX=off  SenseOmegaY=off  SenseOmegaZ=off  SenseQDot=off  SenseRDot=off  SenseAlphaX=off  SenseAlphaY=off  SenseAlphaZ=off  SenseQDDot=off  SenseRDDot=off  SenseX=on  SenseY=on  SenseZ=on  SenseRad=off  SenseAzim=off  SenseDist=off  SenseInc=off  SenseXDot=on  SenseYDot=on  SenseZDot=on  SenseRadDot=off  SenseAzimDot=off  SenseDistDot=off  SenseIncDot=off  SenseXDDot=off  SenseYDDot=off  SenseZDDot=off  SenseRadDDot=off  SenseAzimDDot=off  SenseDistDDot=off  SenseIncDDot=off
  PS-Simulink Converter{1..3,13..15} (6 alike) : nesl_utility/PS-Simulink Converter  PhysicalDomain=network_engine_domain  SubClassName=ps_output  LeftPortType=input  RightPortType=output  PseudoPeriodic=off  Frequencies=[]  VectorFormat=inherit  Unit=inherit  AffineConversion=off
  Vector Concatenate1 : Concatenate  NumInputs=3
  Vector Concatenate3 : Concatenate  NumInputs=3
  B : PMIOPort  Side=Left
  F : PMIOPort  Port=2  Side=Left
  p : Outport
  v : Outport  Port=2
  wires:
  PS-Simulink Converter13/1 -> Vector Concatenate3/1
  PS-Simulink Converter15/1 -> Vector Concatenate3/3
  PS-Simulink Converter14/1 -> Vector Concatenate3/2
  Vector Concatenate3/1 -> p/1
  PS-Simulink Converter2/1 -> Vector Concatenate1/2
  PS-Simulink Converter3/1 -> Vector Concatenate1/3
  PS-Simulink Converter1/1 -> Vector Concatenate1/1
  Vector Concatenate1/1 -> v/1
  connections:
  FootPos_FL/LConn1 -- B-frame/RConn1 -- B/RConn1
  FootPos_FL/RConn1 -- F-frame/RConn1 -- F/RConn1
  FootPos_FL/RConn4 -- PS-Simulink Converter15/LConn1
  FootPos_FL/RConn2 -- PS-Simulink Converter13/LConn1
  FootPos_FL/RConn3 -- PS-Simulink Converter14/LConn1
  FootPos_FL/RConn6 -- PS-Simulink Converter2/LConn1
  FootPos_FL/RConn5 -- PS-Simulink Converter1/LConn1
  FootPos_FL/RConn7 -- PS-Simulink Converter3/LConn1

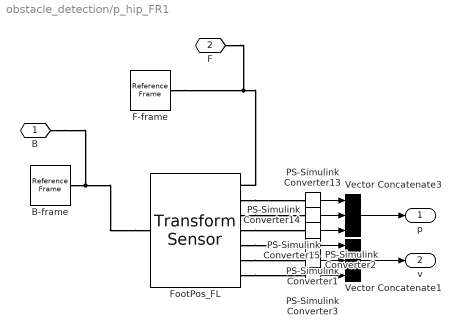
== system obstacle_detection/p_hip_FR1 ==
  B-frame : sm_lib/Frames and Transforms/Reference Frame
  F-frame : sm_lib/Frames and Transforms/Reference Frame
  FootPos_FL : sm_lib/Frames and Transforms/Transform Sensor  MeasurementFrame=World  SenseAngle=off  SenseAxis=off  SenseQ=off  SenseR=off  SenseRotationSequence=off  RotationSequence=XYX  SenseOmegaX=off  SenseOmegaY=off  SenseOmegaZ=off  SenseQDot=off  SenseRDot=off  SenseAlphaX=off  SenseAlphaY=off  SenseAlphaZ=off  SenseQDDot=off  SenseRDDot=off  SenseX=on  SenseY=on  SenseZ=on  SenseRad=off  SenseAzim=off  SenseDist=off  SenseInc=off  SenseXDot=on  SenseYDot=on  SenseZDot=on  SenseRadDot=off  SenseAzimDot=off  SenseDistDot=off  SenseIncDot=off  SenseXDDot=off  SenseYDDot=off  SenseZDDot=off  SenseRadDDot=off  SenseAzimDDot=off  SenseDistDDot=off  SenseIncDDot=off
  PS-Simulink Converter{1..3,13..15} (6 alike) : nesl_utility/PS-Simulink Converter  PhysicalDomain=network_engine_domain  SubClassName=ps_output  LeftPortType=input  RightPortType=output  PseudoPeriodic=off  Frequencies=[]  VectorFormat=inherit  Unit=inherit  AffineConversion=off
  Vector Concatenate1 : Concatenate  NumInputs=3
  Vector Concatenate3 : Concatenate  NumInputs=3
  B : PMIOPort  Side=Left
  F : PMIOPort  Port=2  Side=Left
  p : Outport
  v : Outport  Port=2
  wires:
  PS-Simulink Converter13/1 -> Vector Concatenate3/1
  PS-Simulink Converter15/1 -> Vector Concatenate3/3
  PS-Simulink Converter14/1 -> Vector Concatenate3/2
  Vector Concatenate3/1 -> p/1
  PS-Simulink Converter2/1 -> Vector Concatenate1/2
  PS-Simulink Converter3/1 -> Vector Concatenate1/3
  PS-Simulink Converter1/1 -> Vector Concatenate1/1
  Vector Concatenate1/1 -> v/1
  connections:
  FootPos_FL/LConn1 -- B-frame/RConn1 -- B/RConn1
  FootPos_FL/RConn1 -- F-frame/RConn1 -- F/RConn1
  FootPos_FL/RConn4 -- PS-Simulink Converter15/LConn1
  FootPos_FL/RConn2 -- PS-Simulink Converter13/LConn1
  FootPos_FL/RConn3 -- PS-Simulink Converter14/LConn1
  FootPos_FL/RConn6 -- PS-Simulink Converter2/LConn1
  FootPos_FL/RConn5 -- PS-Simulink Converter1/LConn1
  FootPos_FL/RConn7 -- PS-Simulink Converter3/LConn1

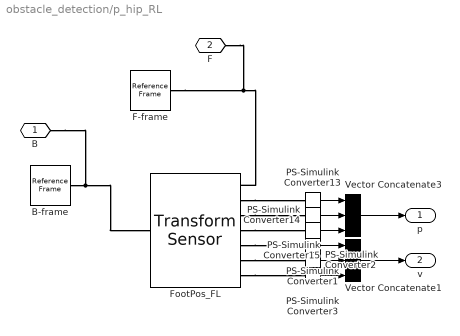
== system obstacle_detection/p_hip_RL ==
  B-frame : sm_lib/Frames and Transforms/Reference Frame
  F-frame : sm_lib/Frames and Transforms/Reference Frame
  FootPos_FL : sm_lib/Frames and Transforms/Transform Sensor  MeasurementFrame=World  SenseAngle=off  SenseAxis=off  SenseQ=off  SenseR=off  SenseRotationSequence=off  RotationSequence=XYX  SenseOmegaX=off  SenseOmegaY=off  SenseOmegaZ=off  SenseQDot=off  SenseRDot=off  SenseAlphaX=off  SenseAlphaY=off  SenseAlphaZ=off  SenseQDDot=off  SenseRDDot=off  SenseX=on  SenseY=on  SenseZ=on  SenseRad=off  SenseAzim=off  SenseDist=off  SenseInc=off  SenseXDot=on  SenseYDot=on  SenseZDot=on  SenseRadDot=off  SenseAzimDot=off  SenseDistDot=off  SenseIncDot=off  SenseXDDot=off  SenseYDDot=off  SenseZDDot=off  SenseRadDDot=off  SenseAzimDDot=off  SenseDistDDot=off  SenseIncDDot=off
  PS-Simulink Converter{1..3,13..15} (6 alike) : nesl_utility/PS-Simulink Converter  PhysicalDomain=network_engine_domain  SubClassName=ps_output  LeftPortType=input  RightPortType=output  PseudoPeriodic=off  Frequencies=[]  VectorFormat=inherit  Unit=inherit  AffineConversion=off
  Vector Concatenate1 : Concatenate  NumInputs=3
  Vector Concatenate3 : Concatenate  NumInputs=3
  B : PMIOPort  Side=Left
  F : PMIOPort  Port=2  Side=Left
  p : Outport
  v : Outport  Port=2
  wires:
  Vector Concatenate1/1 -> v/1
  PS-Simulink Converter1/1 -> Vector Concatenate1/1
  PS-Simulink Converter3/1 -> Vector Concatenate1/3
  PS-Simulink Converter2/1 -> Vector Concatenate1/2
  Vector Concatenate3/1 -> p/1
  PS-Simulink Converter14/1 -> Vector Concatenate3/2
  PS-Simulink Converter15/1 -> Vector Concatenate3/3
  PS-Simulink Converter13/1 -> Vector Concatenate3/1
  connections:
  FootPos_FL/RConn7 -- PS-Simulink Converter3/LConn1
  FootPos_FL/RConn5 -- PS-Simulink Converter1/LConn1
  FootPos_FL/RConn6 -- PS-Simulink Converter2/LConn1
  FootPos_FL/RConn3 -- PS-Simulink Converter14/LConn1
  FootPos_FL/RConn2 -- PS-Simulink Converter13/LConn1
  FootPos_FL/RConn4 -- PS-Simulink Converter15/LConn1
  F/RConn1 -- F-frame/RConn1 -- FootPos_FL/RConn1
  B/RConn1 -- B-frame/RConn1 -- FootPos_FL/LConn1

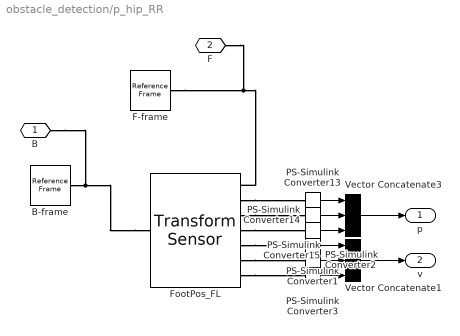
== system obstacle_detection/p_hip_RR ==
  B-frame : sm_lib/Frames and Transforms/Reference Frame
  F-frame : sm_lib/Frames and Transforms/Reference Frame
  FootPos_FL : sm_lib/Frames and Transforms/Transform Sensor  MeasurementFrame=World  SenseAngle=off  SenseAxis=off  SenseQ=off  SenseR=off  SenseRotationSequence=off  RotationSequence=XYX  SenseOmegaX=off  SenseOmegaY=off  SenseOmegaZ=off  SenseQDot=off  SenseRDot=off  SenseAlphaX=off  SenseAlphaY=off  SenseAlphaZ=off  SenseQDDot=off  SenseRDDot=off  SenseX=on  SenseY=on  SenseZ=on  SenseRad=off  SenseAzim=off  SenseDist=off  SenseInc=off  SenseXDot=on  SenseYDot=on  SenseZDot=on  SenseRadDot=off  SenseAzimDot=off  SenseDistDot=off  SenseIncDot=off  SenseXDDot=off  SenseYDDot=off  SenseZDDot=off  SenseRadDDot=off  SenseAzimDDot=off  SenseDistDDot=off  SenseIncDDot=off
  PS-Simulink Converter{1..3,13..15} (6 alike) : nesl_utility/PS-Simulink Converter  PhysicalDomain=network_engine_domain  SubClassName=ps_output  LeftPortType=input  RightPortType=output  PseudoPeriodic=off  Frequencies=[]  VectorFormat=inherit  Unit=inherit  AffineConversion=off
  Vector Concatenate1 : Concatenate  NumInputs=3
  Vector Concatenate3 : Concatenate  NumInputs=3
  B : PMIOPort  Side=Left
  F : PMIOPort  Port=2  Side=Left
  p : Outport
  v : Outport  Port=2
  wires:
  PS-Simulink Converter13/1 -> Vector Concatenate3/1
  PS-Simulink Converter15/1 -> Vector Concatenate3/3
  PS-Simulink Converter14/1 -> Vector Concatenate3/2
  Vector Concatenate3/1 -> p/1
  PS-Simulink Converter2/1 -> Vector Concatenate1/2
  PS-Simulink Converter3/1 -> Vector Concatenate1/3
  PS-Simulink Converter1/1 -> Vector Concatenate1/1
  Vector Concatenate1/1 -> v/1
  connections:
  FootPos_FL/LConn1 -- B-frame/RConn1 -- B/RConn1
  FootPos_FL/RConn1 -- F-frame/RConn1 -- F/RConn1
  FootPos_FL/RConn4 -- PS-Simulink Converter15/LConn1
  FootPos_FL/RConn2 -- PS-Simulink Converter13/LConn1
  FootPos_FL/RConn3 -- PS-Simulink Converter14/LConn1
  FootPos_FL/RConn6 -- PS-Simulink Converter2/LConn1
  FootPos_FL/RConn5 -- PS-Simulink Converter1/LConn1
  FootPos_FL/RConn7 -- PS-Simulink Converter3/LConn1

== system obstacle_detection/pv_FL_foot ==
  B-frame : sm_lib/Frames and Transforms/Reference Frame
  F-frame : sm_lib/Frames and Transforms/Reference Frame
  FootPos_FL : sm_lib/Frames and Transforms/Transform Sensor  MeasurementFrame=World  SenseAngle=off  SenseAxis=off  SenseQ=off  SenseR=off  SenseRotationSequence=off  RotationSequence=XYX  SenseOmegaX=off  SenseOmegaY=off  SenseOmegaZ=off  SenseQDot=off  SenseRDot=off  SenseAlphaX=off  SenseAlphaY=off  SenseAlphaZ=off  SenseQDDot=off  SenseRDDot=off  SenseX=on  SenseY=on  SenseZ=on  SenseRad=off  SenseAzim=off  SenseDist=off  SenseInc=off  SenseXDot=on  SenseYDot=on  SenseZDot=on  SenseRadDot=off  SenseAzimDot=off  SenseDistDot=off  SenseIncDot=off  SenseXDDot=off  SenseYDDot=off  SenseZDDot=off  SenseRadDDot=off  SenseAzimDDot=off  SenseDistDDot=off  SenseIncDDot=off
  PS-Simulink Converter{1..3,13..15} (6 alike) : nesl_utility/PS-Simulink Converter  PhysicalDomain=network_engine_domain  SubClassName=ps_output  LeftPortType=input  RightPortType=output  PseudoPeriodic=off  Frequencies=[]  VectorFormat=inherit  Unit=inherit  AffineConversion=off
  Vector Concatenate1 : Concatenate  NumInputs=3
  Vector Concatenate3 : Concatenate  NumInputs=3
  B : PMIOPort  Side=Left
  F : PMIOPort  Port=2  Side=Left
  p : Outport
  v : Outport  Port=2
  wires:
  PS-Simulink Converter13/1 -> Vector Concatenate3/1
  PS-Simulink Converter15/1 -> Vector Concatenate3/3
  PS-Simulink Converter14/1 -> Vector Concatenate3/2
  Vector Concatenate3/1 -> p/1
  PS-Simulink Converter2/1 -> Vector Concatenate1/2
  PS-Simulink Converter3/1 -> Vector Concatenate1/3
  PS-Simulink Converter1/1 -> Vector Concatenate1/1
  Vector Concatenate1/1 -> v/1
  connections:
  B-frame/RConn1 -- B/RConn1 -- FootPos_FL/LConn1
  F-frame/RConn1 -- F/RConn1 -- FootPos_FL/RConn1
  FootPos_FL/RConn4 -- PS-Simulink Converter15/LConn1
  FootPos_FL/RConn2 -- PS-Simulink Converter13/LConn1
  FootPos_FL/RConn3 -- PS-Simulink Converter14/LConn1
  FootPos_FL/RConn6 -- PS-Simulink Converter2/LConn1
  FootPos_FL/RConn5 -- PS-Simulink Converter1/LConn1
  FootPos_FL/RConn7 -- PS-Simulink Converter3/LConn1

== system obstacle_detection/pv_FR_foot ==
  B-frame : sm_lib/Frames and Transforms/Reference Frame
  F-frame : sm_lib/Frames and Transforms/Reference Frame
  FootPos_FL : sm_lib/Frames and Transforms/Transform Sensor  MeasurementFrame=World  SenseAngle=off  SenseAxis=off  SenseQ=off  SenseR=off  SenseRotationSequence=off  RotationSequence=XYX  SenseOmegaX=off  SenseOmegaY=off  SenseOmegaZ=off  SenseQDot=off  SenseRDot=off  SenseAlphaX=off  SenseAlphaY=off  SenseAlphaZ=off  SenseQDDot=off  SenseRDDot=off  SenseX=on  SenseY=on  SenseZ=on  SenseRad=off  SenseAzim=off  SenseDist=off  SenseInc=off  SenseXDot=on  SenseYDot=on  SenseZDot=on  SenseRadDot=off  SenseAzimDot=off  SenseDistDot=off  SenseIncDot=off  SenseXDDot=off  SenseYDDot=off  SenseZDDot=off  SenseRadDDot=off  SenseAzimDDot=off  SenseDistDDot=off  SenseIncDDot=off
  PS-Simulink Converter{1..3,13..15} (6 alike) : nesl_utility/PS-Simulink Converter  PhysicalDomain=network_engine_domain  SubClassName=ps_output  LeftPortType=input  RightPortType=output  PseudoPeriodic=off  Frequencies=[]  VectorFormat=inherit  Unit=inherit  AffineConversion=off
  Vector Concatenate1 : Concatenate  NumInputs=3
  Vector Concatenate3 : Concatenate  NumInputs=3
  B : PMIOPort  Side=Left
  F : PMIOPort  Port=2  Side=Left
  p : Outport
  v : Outport  Port=2
  wires:
  PS-Simulink Converter13/1 -> Vector Concatenate3/1
  PS-Simulink Converter15/1 -> Vector Concatenate3/3
  PS-Simulink Converter14/1 -> Vector Concatenate3/2
  Vector Concatenate3/1 -> p/1
  PS-Simulink Converter2/1 -> Vector Concatenate1/2
  PS-Simulink Converter3/1 -> Vector Concatenate1/3
  PS-Simulink Converter1/1 -> Vector Concatenate1/1
  Vector Concatenate1/1 -> v/1
  connections:
  FootPos_FL/LConn1 -- B-frame/RConn1 -- B/RConn1
  FootPos_FL/RConn1 -- F-frame/RConn1 -- F/RConn1
  FootPos_FL/RConn4 -- PS-Simulink Converter15/LConn1
  FootPos_FL/RConn2 -- PS-Simulink Converter13/LConn1
  FootPos_FL/RConn3 -- PS-Simulink Converter14/LConn1
  FootPos_FL/RConn6 -- PS-Simulink Converter2/LConn1
  FootPos_FL/RConn5 -- PS-Simulink Converter1/LConn1
  FootPos_FL/RConn7 -- PS-Simulink Converter3/LConn1

== system obstacle_detection/pv_RL_foot ==
  B-frame : sm_lib/Frames and Transforms/Reference Frame
  F-frame : sm_lib/Frames and Transforms/Reference Frame
  FootPos_FL : sm_lib/Frames and Transforms/Transform Sensor  MeasurementFrame=World  SenseAngle=off  SenseAxis=off  SenseQ=off  SenseR=off  SenseRotationSequence=off  RotationSequence=XYX  SenseOmegaX=off  SenseOmegaY=off  SenseOmegaZ=off  SenseQDot=off  SenseRDot=off  SenseAlphaX=off  SenseAlphaY=off  SenseAlphaZ=off  SenseQDDot=off  SenseRDDot=off  SenseX=on  SenseY=on  SenseZ=on  SenseRad=off  SenseAzim=off  SenseDist=off  SenseInc=off  SenseXDot=on  SenseYDot=on  SenseZDot=on  SenseRadDot=off  SenseAzimDot=off  SenseDistDot=off  SenseIncDot=off  SenseXDDot=off  SenseYDDot=off  SenseZDDot=off  SenseRadDDot=off  SenseAzimDDot=off  SenseDistDDot=off  SenseIncDDot=off
  PS-Simulink Converter{1..3,13..15} (6 alike) : nesl_utility/PS-Simulink Converter  PhysicalDomain=network_engine_domain  SubClassName=ps_output  LeftPortType=input  RightPortType=output  PseudoPeriodic=off  Frequencies=[]  VectorFormat=inherit  Unit=inherit  AffineConversion=off
  Vector Concatenate1 : Concatenate  NumInputs=3
  Vector Concatenate3 : Concatenate  NumInputs=3
  B : PMIOPort  Side=Left
  F : PMIOPort  Port=2  Side=Left
  p : Outport
  v : Outport  Port=2
  wires:
  Vector Concatenate1/1 -> v/1
  PS-Simulink Converter1/1 -> Vector Concatenate1/1
  PS-Simulink Converter3/1 -> Vector Concatenate1/3
  PS-Simulink Converter2/1 -> Vector Concatenate1/2
  Vector Concatenate3/1 -> p/1
  PS-Simulink Converter14/1 -> Vector Concatenate3/2
  PS-Simulink Converter15/1 -> Vector Concatenate3/3
  PS-Simulink Converter13/1 -> Vector Concatenate3/1
  connections:
  FootPos_FL/RConn7 -- PS-Simulink Converter3/LConn1
  FootPos_FL/RConn5 -- PS-Simulink Converter1/LConn1
  FootPos_FL/RConn6 -- PS-Simulink Converter2/LConn1
  FootPos_FL/RConn3 -- PS-Simulink Converter14/LConn1
  FootPos_FL/RConn2 -- PS-Simulink Converter13/LConn1
  FootPos_FL/RConn4 -- PS-Simulink Converter15/LConn1
  F/RConn1 -- F-frame/RConn1 -- FootPos_FL/RConn1
  B/RConn1 -- B-frame/RConn1 -- FootPos_FL/LConn1

== system obstacle_detection/pv_RR_foot ==
  B-frame : sm_lib/Frames and Transforms/Reference Frame
  F-frame : sm_lib/Frames and Transforms/Reference Frame
  FootPos_FL : sm_lib/Frames and Transforms/Transform Sensor  MeasurementFrame=World  SenseAngle=off  SenseAxis=off  SenseQ=off  SenseR=off  SenseRotationSequence=off  RotationSequence=XYX  SenseOmegaX=off  SenseOmegaY=off  SenseOmegaZ=off  SenseQDot=off  SenseRDot=off  SenseAlphaX=off  SenseAlphaY=off  SenseAlphaZ=off  SenseQDDot=off  SenseRDDot=off  SenseX=on  SenseY=on  SenseZ=on  SenseRad=off  SenseAzim=off  SenseDist=off  SenseInc=off  SenseXDot=on  SenseYDot=on  SenseZDot=on  SenseRadDot=off  SenseAzimDot=off  SenseDistDot=off  SenseIncDot=off  SenseXDDot=off  SenseYDDot=off  SenseZDDot=off  SenseRadDDot=off  SenseAzimDDot=off  SenseDistDDot=off  SenseIncDDot=off
  PS-Simulink Converter{1..3,13..15} (6 alike) : nesl_utility/PS-Simulink Converter  PhysicalDomain=network_engine_domain  SubClassName=ps_output  LeftPortType=input  RightPortType=output  PseudoPeriodic=off  Frequencies=[]  VectorFormat=inherit  Unit=inherit  AffineConversion=off
  Vector Concatenate1 : Concatenate  NumInputs=3
  Vector Concatenate3 : Concatenate  NumInputs=3
  B : PMIOPort  Side=Left
  F : PMIOPort  Port=2  Side=Left
  p : Outport
  v : Outport  Port=2
  wires:
  PS-Simulink Converter13/1 -> Vector Concatenate3/1
  PS-Simulink Converter15/1 -> Vector Concatenate3/3
  PS-Simulink Converter14/1 -> Vector Concatenate3/2
  Vector Concatenate3/1 -> p/1
  PS-Simulink Converter2/1 -> Vector Concatenate1/2
  PS-Simulink Converter3/1 -> Vector Concatenate1/3
  PS-Simulink Converter1/1 -> Vector Concatenate1/1
  Vector Concatenate1/1 -> v/1
  connections:
  FootPos_FL/LConn1 -- B-frame/RConn1 -- B/RConn1
  FootPos_FL/RConn1 -- F-frame/RConn1 -- F/RConn1
  FootPos_FL/RConn4 -- PS-Simulink Converter15/LConn1
  FootPos_FL/RConn2 -- PS-Simulink Converter13/LConn1
  FootPos_FL/RConn3 -- PS-Simulink Converter14/LConn1
  FootPos_FL/RConn6 -- PS-Simulink Converter2/LConn1
  FootPos_FL/RConn5 -- PS-Simulink Converter1/LConn1
  FootPos_FL/RConn7 -- PS-Simulink Converter3/LConn1

== system obstacle_detection/q ==
  RR_calf : Inport
  RL_calf : Inport  Port=2
  FR_calf : Inport  Port=3
  FL_calf : Inport  Port=4
  RR_thigh : Inport  Port=5
  RL_thigh : Inport  Port=6
  FR_thigh : Inport  Port=7
  FL_thigh : Inport  Port=8
  RR_hip : Inport  Port=9
  RL_hip : Inport  Port=10
  FR_hip : Inport  Port=11
  FL_hip : Inport  Port=12
  Joint Angles : Scope  NumInputPorts=12
  Vector Concatenate : Concatenate  NumInputs=12
  joint vector : Outport
  wires:
  RR_calf/1 -> Joint Angles/1, Vector Concatenate/1
  RL_calf/1 -> Joint Angles/2, Vector Concatenate/2
  FR_calf/1 -> Joint Angles/3, Vector Concatenate/3
  FL_calf/1 -> Joint Angles/4, Vector Concatenate/4
  RR_thigh/1 -> Joint Angles/5, Vector Concatenate/5
  RL_thigh/1 -> Vector Concatenate/6, Joint Angles/6
  FR_thigh/1 -> Vector Concatenate/7, Joint Angles/7
  FL_thigh/1 -> Joint Angles/8, Vector Concatenate/8
  RR_hip/1 -> Joint Angles/9, Vector Concatenate/9
  RL_hip/1 -> Joint Angles/10, Vector Concatenate/10
  FR_hip/1 -> Joint Angles/11, Vector Concatenate/11
  FL_hip/1 -> Joint Angles/12, Vector Concatenate/12
  Vector Concatenate/1 -> joint vector/1
